simulink model "Question_5"  (R2024b)
settings: Solver=VariableStepAuto  StartTime=0.0  StopTime=10.0  RelTol=1e-3
model workspace (MAT data in the model file):
  b1 = 1
  b2 = 1
  b3 = 1
  k1 = 3
  k2 = 1
  k3 = 1
  m1 = 40
  m2 = 20
  m3 = 10
  u1 = 10
  u2 = 10
  u3 = 10
settings Model: Creator=Sagar  LastModifiedBy=Sagar

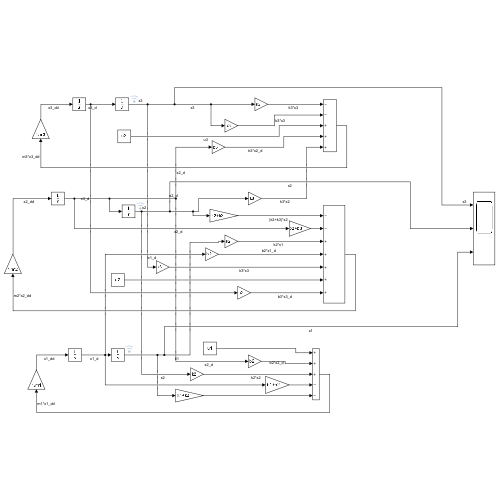
[thumbnail: Simulink's stored preview of the top-level diagram]
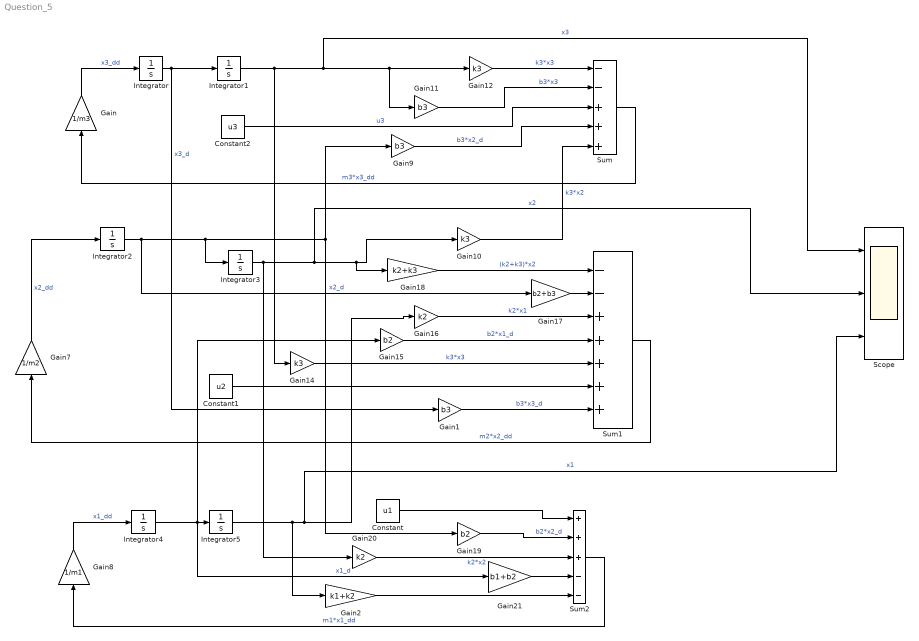
== system Question_5 ==
  Constant : Constant  Value=u1
  Constant1 : Constant  Value=u2
  Constant2 : Constant  Value=u3
  Gain : Gain  Gain=1/m3
  Gain1 : Gain  Gain=b3
  Gain10 : Gain  Gain=k3
  Gain11 : Gain  Gain=b3
  Gain12 : Gain  Gain=k3
  Gain14 : Gain  Gain=k3
  Gain15 : Gain  Gain=b2
  Gain16 : Gain  Gain=k2
  Gain17 : Gain  Gain=b2+b3
  Gain18 : Gain  Gain=k2+k3
  Gain19 : Gain  Gain=b2
  Gain2 : Gain  Gain=k1+k2
  Gain20 : Gain  Gain=k2
  Gain21 : Gain  Gain=b1+b2
  Gain7 : Gain  Gain=1/m2
  Gain8 : Gain  Gain=1/m1
  Gain9 : Gain  Gain=b3
  Integrator{,1..5} (6 alike) : Integrator
  Scope : Scope  NumInputPorts=3
  Sum : Sum  Inputs=--+++
  Sum1 : Sum  Inputs=--+++++
  Sum2 : Sum  Inputs=+++--
  wires:
  Gain/1 -> Integrator/1  "x3_dd"
  Integrator/1 -> Integrator1/1, Gain1/1  "x3_d"
  Integrator1/1 -> Scope/1, Gain11/1, Gain12/1, Gain14/1  "x3"
  Sum/1 -> Gain/1  "m3*x3_dd"
  Sum1/1 -> Gain7/1  "m2*x2_dd"
  Integrator3/1 -> Scope/2, Gain10/1, Gain18/1, Gain20/1  "x2"
  Integrator2/1 -> Integrator3/1, Gain19/1, Gain9/1, Gain17/1  "x2_d"
  Gain7/1 -> Integrator2/1  "x2_dd"
  Gain8/1 -> Integrator4/1  "x1_dd"
  Integrator4/1 -> Gain15/1, Integrator5/1, Gain21/1  "x1_d"
  Integrator5/1 -> Gain2/1, Scope/3, Gain16/1  "x1"
  Sum2/1 -> Gain8/1  "m1*x1_dd"
  Gain9/1 -> Sum/4  "b3*x2_d"
  Constant2/1 -> Sum/3  "u3"
  Gain10/1 -> Sum/5  "k3*x2"
  Gain11/1 -> Sum/2  "b3*x3"
  Gain12/1 -> Sum/1  "k3*x3"
  Constant1/1 -> Sum1/6
  Gain1/1 -> Sum1/7  "b3*x3_d"
  Gain14/1 -> Sum1/5  "k3*x3"
  Gain15/1 -> Sum1/4  "b2*x1_d"
  Gain16/1 -> Sum1/3  "k2*x1"
  Gain17/1 -> Sum1/2
  Gain18/1 -> Sum1/1  "(k2+k3)*x2"
  Constant/1 -> Sum2/1
  Gain19/1 -> Sum2/2  "b2*x2_d"
  Gain20/1 -> Sum2/3  "k2*x2"
  Gain21/1 -> Sum2/4
  Gain2/1 -> Sum2/5
